simulink model "TrajectoryControl"  (R2020b)
settings: Solver=ode3  StartTime=0.0  StopTime=100.0  FixedStep=Ts  RelTol=1e-3
values from neighbouring files (symbols this model uses):
  th_0 = 0    [Ejercicio2.m]
  Ts = 100e-3    (= 0.1)    [Ejercicio1.m]    (also in Ejercicio2.m)
  x_0 = 0.02    [Ejercicio2.m]
  y_0 = 0    [Ejercicio2.m]
undefined symbols (not defined in the file or in its folder): DiscIntNeverNeededParam, sigbuilder_block
libraries: simulink x1, fuzblock x1
settings Model: Creator=patri  LastModifiedBy=patri
settings DataIOCC: ReturnWorkspaceOutputs=off

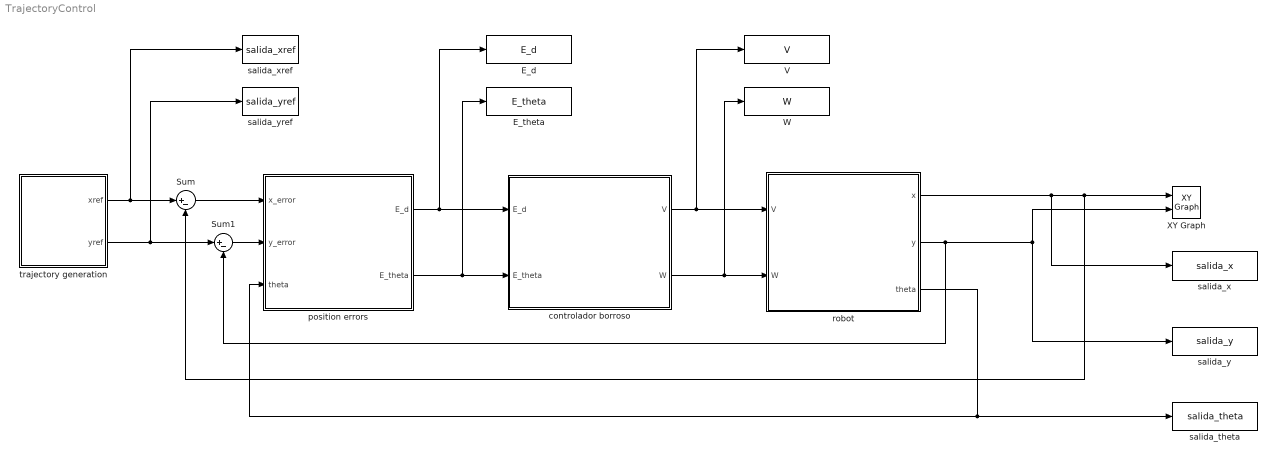
== system TrajectoryControl ==
  E_d : ToWorkspace  VariableName=E_d  SaveFormat=Structure With Time  SampleTime=-1
  E_theta : ToWorkspace  VariableName=E_theta  SaveFormat=Structure With Time  SampleTime=-1
  Sum : Sum  Inputs=|+-
  Sum1 : Sum  Inputs=|+-
  V : ToWorkspace  VariableName=V  SaveFormat=Structure With Time  SampleTime=-1
  W : ToWorkspace  VariableName=W  SaveFormat=Structure With Time  SampleTime=-1
  XY Graph : simulink/Sinks/XY Graph  xmin=-20  xmax=20  ymin=-20  ymax=20  st=-1
  controlador borroso : Subsystem
  position errors : Subsystem
  robot : Subsystem
  salida_theta : ToWorkspace  VariableName=salida_theta  SaveFormat=Structure With Time  SampleTime=-1
  salida_x : ToWorkspace  VariableName=salida_x  SaveFormat=Structure With Time  SampleTime=-1
  salida_xref : ToWorkspace  VariableName=salida_xref  SaveFormat=Structure With Time  SampleTime=-1
  salida_y : ToWorkspace  VariableName=salida_y  SaveFormat=Structure With Time  SampleTime=-1
  salida_yref : ToWorkspace  VariableName=salida_yref  SaveFormat=Structure With Time  SampleTime=-1
  trajectory generation : Subsystem
  wires:
  controlador borroso/1(V) -> robot/1(V), V/1
  position errors/1(E_d) -> E_d/1, controlador borroso/1(E_d)
  robot/1(x) -> salida_x/1, Sum/2, XY Graph/1
  controlador borroso/2(W) -> robot/2(W), W/1
  robot/2(y) -> Sum1/2, salida_y/1, XY Graph/2
  robot/3(theta) -> salida_theta/1, position errors/3(theta)
  position errors/2(E_theta) -> E_theta/1, controlador borroso/2(E_theta)
  trajectory generation/1(xref) -> salida_xref/1, Sum/1
  trajectory generation/2(yref) -> salida_yref/1, Sum1/1
  Sum1/1 -> position errors/2(y_error)
  Sum/1 -> position errors/1(x_error)

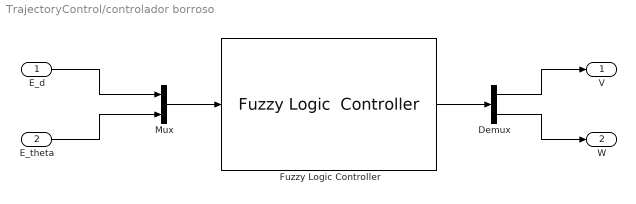
== system TrajectoryControl/controlador borroso ==
  E_d : Inport
  E_theta : Inport  Port=2
  Demux : Demux  Outputs=2
  Fuzzy Logic Controller : fuzblock/Fuzzy Logic  Controller  FIS='ControlBorroso.fis'  OutputSampleNumber=101  DataType=double  FuzzifiedInputs=off  RuleFiringStrengths=off  RuleOutputs=off  AggregatedOutputs=off  SimulateUsing=Interpreted execution  OutOfRangeInputValueMessage=warning  NoRuleFiredMessage=warning  EmptyOutputFuzzySetMessage=warning
  Mux : Mux  Inputs=2
  V : Outport
  W : Outport  Port=2
  wires:
  Mux/1 -> Fuzzy Logic Controller/1
  E_theta/1 -> Mux/2
  Demux/1 -> V/1
  Fuzzy Logic Controller/1 -> Demux/1
  E_d/1 -> Mux/1
  Demux/2 -> W/1

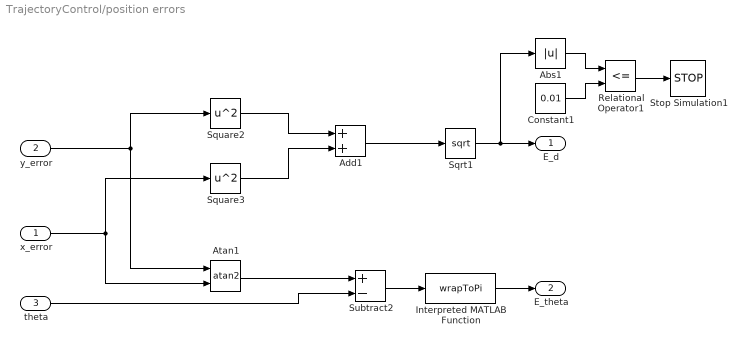
== system TrajectoryControl/position errors ==
  x_error : Inport
  y_error : Inport  Port=2
  theta : Inport  Port=3
  Abs1 : Abs
  Add1 : Sum
  Atan1 : Trigonometry  Operator=atan2
  Constant1 : Constant  Value=0.01
  Interpreted MATLAB Function : MATLABFcn  MATLABFcn=wrapToPi
  Relational Operator1 : RelationalOperator  Operator=<=  OutDataTypeStr=boolean  RndMeth=Simplest
  Sqrt1 : Sqrt  SaturateOnIntegerOverflow=on
  Square2 : Math  Operator=square  SignedPower=on  SaturateOnIntegerOverflow=on
  Square3 : Math  Operator=square  SignedPower=on  SaturateOnIntegerOverflow=on
  Stop Simulation1 : Stop
  Subtract2 : Sum  Inputs=+-  OutMin=[-3.14]  OutMax=[3.14]
  E_d : Outport  VectorParamsAs1DForOutWhenUnconnected=off
  E_theta : Outport  Port=2  OutMin=[-pi]  OutMax=[pi]  VectorParamsAs1DForOutWhenUnconnected=off
  wires:
  Subtract2/1 -> Interpreted MATLAB Function/1
  Relational Operator1/1 -> Stop Simulation1/1
  Atan1/1 -> Subtract2/1
  x_error/1 -> Atan1/2, Square3/1
  Constant1/1 -> Relational Operator1/2
  Interpreted MATLAB Function/1 -> E_theta/1
  Abs1/1 -> Relational Operator1/1
  Square3/1 -> Add1/2
  Sqrt1/1 -> Abs1/1, E_d/1
  Square2/1 -> Add1/1
  Add1/1 -> Sqrt1/1
  theta/1 -> Subtract2/2
  y_error/1 -> Atan1/1, Square2/1

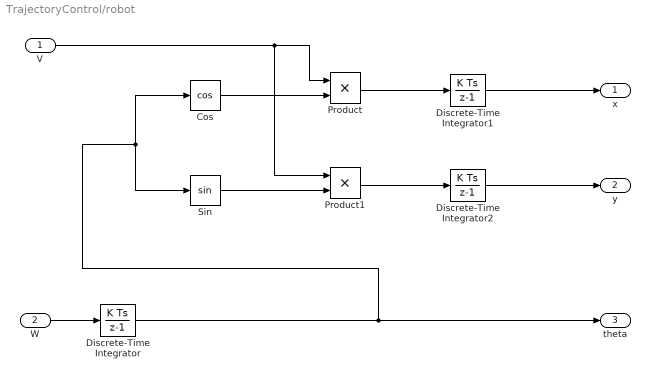
== system TrajectoryControl/robot ==
  V : Inport
  W : Inport  Port=2
  Cos : Trigonometry  Operator=cos
  Discrete-Time Integrator : DiscreteIntegrator  SampleTime=-1  ICPrevOutput=DiscIntNeverNeededParam  ICPrevScaledInput=DiscIntNeverNeededParam
  Discrete-Time Integrator1 : DiscreteIntegrator  SampleTime=-1  ICPrevOutput=DiscIntNeverNeededParam  ICPrevScaledInput=DiscIntNeverNeededParam
  Discrete-Time Integrator2 : DiscreteIntegrator  SampleTime=-1  ICPrevOutput=DiscIntNeverNeededParam  ICPrevScaledInput=DiscIntNeverNeededParam
  Product : Product
  Product1 : Product
  Sin : Trigonometry
  x : Outport  VectorParamsAs1DForOutWhenUnconnected=off
  y : Outport  Port=2  VectorParamsAs1DForOutWhenUnconnected=off
  theta : Outport  Port=3  VectorParamsAs1DForOutWhenUnconnected=off
  wires:
  Discrete-Time Integrator2/1 -> y/1
  W/1 -> Discrete-Time Integrator/1
  Discrete-Time Integrator1/1 -> x/1
  Discrete-Time Integrator/1 -> theta/1, Sin/1, Cos/1
  Product1/1 -> Discrete-Time Integrator2/1
  Sin/1 -> Product1/2
  V/1 -> Product1/1, Product/1
  Product/1 -> Discrete-Time Integrator1/1
  Cos/1 -> Product/2

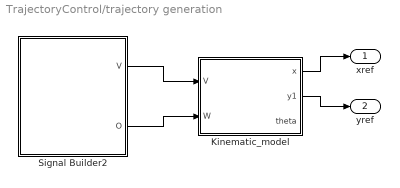
== system TrajectoryControl/trajectory generation ==
  Kinematic_model : Subsystem
  Signal Builder2 : Subsystem  Tag=STV Subsys  LoadFcn=sigbuilder_block('load');  StartFcn=sigbuilder_block('start');  StopFcn=sigbuilder_block('stop');  ClipboardFcn=sigbuilder_block('clipboard');  mask(Sigbuilder block){tuvar=[0:10]}
      mask help: Sigbuilder GUI
      mask init:
      | if ~strcmp(get_param(bdroot(gcbh),'SimulationStatus'),'stopped') tuvar = sigbuilder_block('maskInit'); end
      settings: CopyFcn=sigbuilder_block('copy');  DeleteFcn=sigbuilder_block('delete');  ModelCloseFcn=sigbuilder_block('modelClose');  PreSaveFcn=sigbuilder_block('preSave');  PauseFcn=sigbuilder_block('pause')  ContinueFcn=sigbuilder_block('continue')  NameChangeFcn=sigbuilder_block('namechange');  OpenFcn=sigbuilder_block('open',[60 82.4 534.4 508 ]);  CloseFcn=sigbuilder_block('close');
      mask Display: plot(0, 0, 100, 100,[2, 2, 32, 32, 2], [68, 8, 8, 68, 68],[32, 2], [38, 38], [32, 19, 2],[53, 60, 44], [32, 17, 17, 2],[16, 16, 31, 31]);txt = getActiveGroup(gcbh);text(2, 100, txt,'verticalAlignment', 'top');
  xref : Outport  VectorParamsAs1DForOutWhenUnconnected=off
  yref : Outport  Port=2  VectorParamsAs1DForOutWhenUnconnected=off
  wires:
  Signal Builder2/1(V) -> Kinematic_model/1(V)
  Signal Builder2/2(O) -> Kinematic_model/2("W ")
  Kinematic_model/2(y1) -> yref/1
  Kinematic_model/1("x ") -> xref/1

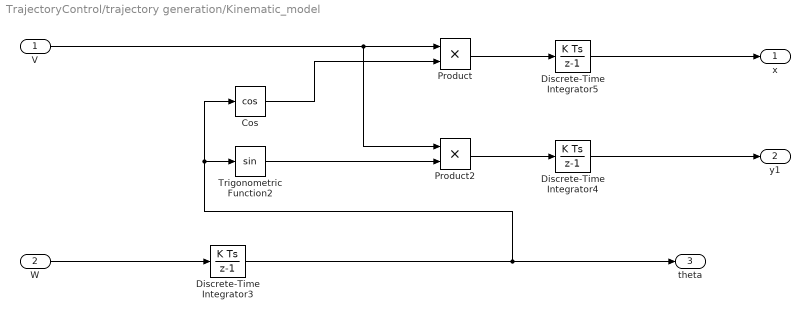
== system TrajectoryControl/trajectory generation/Kinematic_model ==
  V : Inport
  "W " : Inport  Port=2
  Cos : Trigonometry  Operator=cos
  Discrete-Time Integrator3 : DiscreteIntegrator  InitialCondition=th_0  SampleTime=Ts  ICPrevOutput=DiscIntNeverNeededParam  ICPrevScaledInput=DiscIntNeverNeededParam
  Discrete-Time Integrator4 : DiscreteIntegrator  InitialCondition=y_0  SampleTime=Ts  ICPrevOutput=DiscIntNeverNeededParam  ICPrevScaledInput=DiscIntNeverNeededParam
  Discrete-Time Integrator5 : DiscreteIntegrator  InitialCondition=x_0  SampleTime=Ts  ICPrevOutput=DiscIntNeverNeededParam  ICPrevScaledInput=DiscIntNeverNeededParam
  Product : Product
  Product2 : Product
  Trigonometric Function2 : Trigonometry
  "x " : Outport
  y1 : Outport  Port=2
  theta : Outport  Port=3
  wires:
  Product/1 -> Discrete-Time Integrator5/1
  Discrete-Time Integrator5/1 -> "x "/1
  V/1 -> Product2/1, Product/1
  Product2/1 -> Discrete-Time Integrator4/1
  Discrete-Time Integrator3/1 -> theta/1, Cos/1, Trigonometric Function2/1
  Trigonometric Function2/1 -> Product2/2
  "W "/1 -> Discrete-Time Integrator3/1
  Cos/1 -> Product/2
  Discrete-Time Integrator4/1 -> y1/1

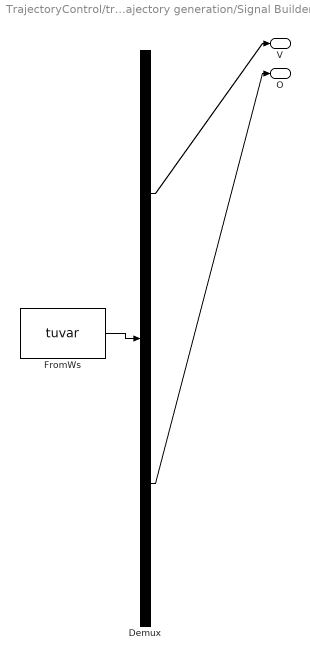
== system TrajectoryControl/trajectory generation/Signal Builder2 ==
  Demux : Demux  Tag=STV Demux  Outputs=2
      settings: DisplayOption=none
  FromWs : FromWorkspace  Tag=STV FromWs  VariableName=tuvar
      SigBuilderData=|
      | common.afterFinalStr = 'Extrapolate'
      | common.sampleTime = '0'
      | dataSet.timeRange = [0 115]
      | dataSet.name = 'Group 1'
      | sbobj.Groups.Name = 'Group 1'
      | sbobj.Groups.Signals(1).Name = 'V'
      | sbobj.Groups.Signals(1).XData = [0 87 87 115]
      | sbobj.Groups.Signals(1).YData = [0.25 0.25 0 0]
      | sbobj.Groups.Signals(2).Name = 'O'
      | sbobj.Groups.Signals(2).XData = [0 12 12 30.849 30.849 55.981 55.981 74.83 74.83 99.962 115]
      | sbobj.Groups.Signals(2).YData = [0 0 0.25 0.25 -0.25 -0.25 0.25 0.25 0 0 0]
      | sbobj.Groups.TimeRange = [0 115]
  V : Outport  Tag=STV Outport  VectorParamsAs1DForOutWhenUnconnected=off
  O : Outport  Tag=STV Outport  Port=2  VectorParamsAs1DForOutWhenUnconnected=off
  wires:
  FromWs/1 -> Demux/1
  Demux/1 -> V/1
  Demux/2 -> O/1
